simulink model "LM_TOS_new"  (R2018b)
settings: Solver=FixedStepDiscrete  StartTime=0.0  StopTime=inf  FixedStep=0.005  RelTol=1e-3
PostLoadFcn:
  | if any(exist('dsrtsu_mdlpostloadfcn', 'file') ~= 0), dsrtsu_mdlpostloadfcn('Execute', bdroot); end
libraries: rtican x35
(part 10 of 11)

== system LM_TOS_new/LM_TOS_MODEL/adapter2/Lane_2/Subsystem13 ==
  <LANE_2_TARGETOBJECT_0_ST> : Inport
  Bus Creator1 : BusCreator  Inputs=7  OutDataTypeStr=Bus: SEGMENT  NonVirtualBus=on
  Bus Selector4 : BusSelector  OutputSignals=coef_arr_f_0,coef_arr_f_1,coef_arr_f_2,coef_arr_f_3,dlowerLimit_f,dupperLimit_f,numOfSegment_un8,available_b,detectedByVideo_b,quality_f
  Vector Concatenate : Concatenate  NumInputs=4
  SEGMENT_ST : Outport  OutDataTypeStr=Bus: SEGMENT
  wires:
  Bus Selector4/6 -> Bus Creator1/3  "<dupperLimit_f>"
  Bus Selector4/7 -> Bus Creator1/4  "<numOfSegment_un8>"
  Bus Selector4/8 -> Bus Creator1/5  "<available_b>"
  Bus Selector4/9 -> Bus Creator1/6  "<detectedByVideo_b>"
  Bus Selector4/10 -> Bus Creator1/7  "<quality_f>"
  Bus Selector4/5 -> Bus Creator1/2  "<dlowerLimit_f>"
  Vector Concatenate/1 -> Bus Creator1/1
  Bus Selector4/4 -> Vector Concatenate/4  "<coef_arr_f_3>"
  Bus Selector4/3 -> Vector Concatenate/3  "<coef_arr_f_2>"
  Bus Selector4/1 -> Vector Concatenate/1  "<coef_arr_f_0>"
  Bus Selector4/2 -> Vector Concatenate/2  "<coef_arr_f_1>"
  <LANE_2_TARGETOBJECT_0_ST>/1 -> Bus Selector4/1
  Bus Creator1/1 -> SEGMENT_ST/1

== system LM_TOS_new/LM_TOS_MODEL/adapter2/Lane_2/Subsystem14 ==
  <LANE_2_TARGETOBJECT_0_ST> : Inport
  Bus Creator1 : BusCreator  Inputs=7  OutDataTypeStr=Bus: SEGMENT  NonVirtualBus=on
  Bus Selector4 : BusSelector  OutputSignals=coef_arr_f_0,coef_arr_f_1,coef_arr_f_2,coef_arr_f_3,dlowerLimit_f,dupperLimit_f,numOfSegment_un8,available_b,detectedByVideo_b,quality_f
  Vector Concatenate : Concatenate  NumInputs=4
  SEGMENT_ST : Outport  OutDataTypeStr=Bus: SEGMENT
  wires:
  Bus Creator1/1 -> SEGMENT_ST/1
  <LANE_2_TARGETOBJECT_0_ST>/1 -> Bus Selector4/1
  Bus Selector4/2 -> Vector Concatenate/2  "<coef_arr_f_1>"
  Bus Selector4/1 -> Vector Concatenate/1  "<coef_arr_f_0>"
  Bus Selector4/3 -> Vector Concatenate/3  "<coef_arr_f_2>"
  Bus Selector4/4 -> Vector Concatenate/4  "<coef_arr_f_3>"
  Vector Concatenate/1 -> Bus Creator1/1
  Bus Selector4/5 -> Bus Creator1/2  "<dlowerLimit_f>"
  Bus Selector4/10 -> Bus Creator1/7  "<quality_f>"
  Bus Selector4/9 -> Bus Creator1/6  "<detectedByVideo_b>"
  Bus Selector4/8 -> Bus Creator1/5  "<available_b>"
  Bus Selector4/7 -> Bus Creator1/4  "<numOfSegment_un8>"
  Bus Selector4/6 -> Bus Creator1/3  "<dupperLimit_f>"

== system LM_TOS_new/LM_TOS_MODEL/adapter2/Lane_2/Subsystem15 ==
  <LANE_2_TARGETOBJECT_0_ST> : Inport
  Bus Creator1 : BusCreator  Inputs=7  OutDataTypeStr=Bus: SEGMENT  NonVirtualBus=on
  Bus Selector4 : BusSelector  OutputSignals=coef_arr_f_0,coef_arr_f_1,coef_arr_f_2,coef_arr_f_3,dlowerLimit_f,dupperLimit_f,numOfSegment_un8,available_b,detectedByVideo_b,quality_f
  Vector Concatenate : Concatenate  NumInputs=4
  SEGMENT_ST : Outport  OutDataTypeStr=Bus: SEGMENT
  wires:
  Bus Selector4/6 -> Bus Creator1/3  "<dupperLimit_f>"
  Bus Selector4/7 -> Bus Creator1/4  "<numOfSegment_un8>"
  Bus Selector4/8 -> Bus Creator1/5  "<available_b>"
  Bus Selector4/9 -> Bus Creator1/6  "<detectedByVideo_b>"
  Bus Selector4/10 -> Bus Creator1/7  "<quality_f>"
  Bus Selector4/5 -> Bus Creator1/2  "<dlowerLimit_f>"
  Vector Concatenate/1 -> Bus Creator1/1
  Bus Selector4/4 -> Vector Concatenate/4  "<coef_arr_f_3>"
  Bus Selector4/3 -> Vector Concatenate/3  "<coef_arr_f_2>"
  Bus Selector4/1 -> Vector Concatenate/1  "<coef_arr_f_0>"
  Bus Selector4/2 -> Vector Concatenate/2  "<coef_arr_f_1>"
  <LANE_2_TARGETOBJECT_0_ST>/1 -> Bus Selector4/1
  Bus Creator1/1 -> SEGMENT_ST/1

== system LM_TOS_new/LM_TOS_MODEL/adapter2/Lane_2/Subsystem2 ==
  <LANE_0_TARGETOBJECT_0_ST> : Inport
  Bus Creator1 : BusCreator  Inputs=9  OutDataTypeStr=Bus: TARGETOBJECT  NonVirtualBus=on
  Bus Selector4 : BusSelector  OutputSignals=dis2EgoLaneCenter,TTC_f,ID_un8,Index_un8,probWithinLane_arr_f_0,probWithinLane_arr_f_1,probWithinLane_arr_f_2,probWithinLane_arr_f_3,probWithinLane_arr_f_4,probCutIn_f,probCutOut_f,overlap_f,trackingTimeWithinLane_f
  Vector Concatenate : Concatenate  NumInputs=5
  TARGRTOBJECTS_ST : Outport  OutDataTypeStr=Bus: TARGETOBJECT
  wires:
  Bus Selector4/4 -> Bus Creator1/4  "<Index_un8>"
  Bus Creator1/1 -> TARGRTOBJECTS_ST/1
  Bus Selector4/3 -> Bus Creator1/3  "<ID_un8>"
  Vector Concatenate/1 -> Bus Creator1/5
  Bus Selector4/7 -> Vector Concatenate/3  "<probWithinLane_arr_f_2>"
  Bus Selector4/1 -> Bus Creator1/1  "<dis2EgoLaneCenter>"
  Bus Selector4/13 -> Bus Creator1/9  "<trackingTimeWithinLane_f>"
  Bus Selector4/6 -> Vector Concatenate/2  "<probWithinLane_arr_f_1>"
  <LANE_0_TARGETOBJECT_0_ST>/1 -> Bus Selector4/1
  Bus Selector4/5 -> Vector Concatenate/1  "<probWithinLane_arr_f_0>"
  Bus Selector4/2 -> Bus Creator1/2  "<TTC_f>"
  Bus Selector4/9 -> Vector Concatenate/5  "<probWithinLane_arr_f_4>"
  Bus Selector4/12 -> Bus Creator1/8  "<overlap_f>"
  Bus Selector4/10 -> Bus Creator1/6  "<probCutIn_f>"
  Bus Selector4/11 -> Bus Creator1/7  "<probCutOut_f>"
  Bus Selector4/8 -> Vector Concatenate/4  "<probWithinLane_arr_f_3>"

== system LM_TOS_new/LM_TOS_MODEL/adapter2/Lane_2/Subsystem3 ==
  <LANE_0_TARGETOBJECT_0_ST> : Inport
  Bus Creator1 : BusCreator  Inputs=9  OutDataTypeStr=Bus: TARGETOBJECT  NonVirtualBus=on
  Bus Selector4 : BusSelector  OutputSignals=dis2EgoLaneCenter,TTC_f,ID_un8,Index_un8,probWithinLane_arr_f_0,probWithinLane_arr_f_1,probWithinLane_arr_f_2,probWithinLane_arr_f_3,probWithinLane_arr_f_4,probCutIn_f,probCutOut_f,overlap_f,trackingTimeWithinLane_f
  Vector Concatenate : Concatenate  NumInputs=5
  TARGRTOBJECTS_ST : Outport  OutDataTypeStr=Bus: TARGETOBJECT
  wires:
  Bus Selector4/8 -> Vector Concatenate/4  "<probWithinLane_arr_f_3>"
  Bus Selector4/11 -> Bus Creator1/7  "<probCutOut_f>"
  Bus Selector4/10 -> Bus Creator1/6  "<probCutIn_f>"
  Bus Selector4/12 -> Bus Creator1/8  "<overlap_f>"
  Bus Selector4/9 -> Vector Concatenate/5  "<probWithinLane_arr_f_4>"
  Bus Selector4/2 -> Bus Creator1/2  "<TTC_f>"
  Bus Selector4/5 -> Vector Concatenate/1  "<probWithinLane_arr_f_0>"
  <LANE_0_TARGETOBJECT_0_ST>/1 -> Bus Selector4/1
  Bus Selector4/6 -> Vector Concatenate/2  "<probWithinLane_arr_f_1>"
  Bus Selector4/13 -> Bus Creator1/9  "<trackingTimeWithinLane_f>"
  Bus Selector4/1 -> Bus Creator1/1  "<dis2EgoLaneCenter>"
  Bus Selector4/7 -> Vector Concatenate/3  "<probWithinLane_arr_f_2>"
  Vector Concatenate/1 -> Bus Creator1/5
  Bus Selector4/3 -> Bus Creator1/3  "<ID_un8>"
  Bus Creator1/1 -> TARGRTOBJECTS_ST/1
  Bus Selector4/4 -> Bus Creator1/4  "<Index_un8>"

== system LM_TOS_new/LM_TOS_MODEL/adapter2/Lane_2/Subsystem4 ==
  <LANE_0_TARGETOBJECT_0_ST> : Inport
  Bus Creator1 : BusCreator  Inputs=9  OutDataTypeStr=Bus: TARGETOBJECT  NonVirtualBus=on
  Bus Selector4 : BusSelector  OutputSignals=dis2EgoLaneCenter,TTC_f,ID_un8,Index_un8,probWithinLane_arr_f_0,probWithinLane_arr_f_1,probWithinLane_arr_f_2,probWithinLane_arr_f_3,probWithinLane_arr_f_4,probCutIn_f,probCutOut_f,overlap_f,trackingTimeWithinLane_f
  Vector Concatenate : Concatenate  NumInputs=5
  TARGRTOBJECTS_ST : Outport  OutDataTypeStr=Bus: TARGETOBJECT
  wires:
  Bus Selector4/4 -> Bus Creator1/4  "<Index_un8>"
  Bus Creator1/1 -> TARGRTOBJECTS_ST/1
  Bus Selector4/3 -> Bus Creator1/3  "<ID_un8>"
  Vector Concatenate/1 -> Bus Creator1/5
  Bus Selector4/7 -> Vector Concatenate/3  "<probWithinLane_arr_f_2>"
  Bus Selector4/1 -> Bus Creator1/1  "<dis2EgoLaneCenter>"
  Bus Selector4/13 -> Bus Creator1/9  "<trackingTimeWithinLane_f>"
  Bus Selector4/6 -> Vector Concatenate/2  "<probWithinLane_arr_f_1>"
  <LANE_0_TARGETOBJECT_0_ST>/1 -> Bus Selector4/1
  Bus Selector4/5 -> Vector Concatenate/1  "<probWithinLane_arr_f_0>"
  Bus Selector4/2 -> Bus Creator1/2  "<TTC_f>"
  Bus Selector4/9 -> Vector Concatenate/5  "<probWithinLane_arr_f_4>"
  Bus Selector4/12 -> Bus Creator1/8  "<overlap_f>"
  Bus Selector4/10 -> Bus Creator1/6  "<probCutIn_f>"
  Bus Selector4/11 -> Bus Creator1/7  "<probCutOut_f>"
  Bus Selector4/8 -> Vector Concatenate/4  "<probWithinLane_arr_f_3>"

== system LM_TOS_new/LM_TOS_MODEL/adapter2/Lane_2/Subsystem5 ==
  <LANE_0_TARGETOBJECT_0_ST> : Inport
  Bus Creator1 : BusCreator  Inputs=9  OutDataTypeStr=Bus: TARGETOBJECT  NonVirtualBus=on
  Bus Selector4 : BusSelector  OutputSignals=dis2EgoLaneCenter,TTC_f,ID_un8,Index_un8,probWithinLane_arr_f_0,probWithinLane_arr_f_1,probWithinLane_arr_f_2,probWithinLane_arr_f_3,probWithinLane_arr_f_4,probCutIn_f,probCutOut_f,overlap_f,trackingTimeWithinLane_f
  Vector Concatenate : Concatenate  NumInputs=5
  TARGRTOBJECTS_ST : Outport  OutDataTypeStr=Bus: TARGETOBJECT
  wires:
  Bus Selector4/8 -> Vector Concatenate/4  "<probWithinLane_arr_f_3>"
  Bus Selector4/11 -> Bus Creator1/7  "<probCutOut_f>"
  Bus Selector4/10 -> Bus Creator1/6  "<probCutIn_f>"
  Bus Selector4/12 -> Bus Creator1/8  "<overlap_f>"
  Bus Selector4/9 -> Vector Concatenate/5  "<probWithinLane_arr_f_4>"
  Bus Selector4/2 -> Bus Creator1/2  "<TTC_f>"
  Bus Selector4/5 -> Vector Concatenate/1  "<probWithinLane_arr_f_0>"
  <LANE_0_TARGETOBJECT_0_ST>/1 -> Bus Selector4/1
  Bus Selector4/6 -> Vector Concatenate/2  "<probWithinLane_arr_f_1>"
  Bus Selector4/13 -> Bus Creator1/9  "<trackingTimeWithinLane_f>"
  Bus Selector4/1 -> Bus Creator1/1  "<dis2EgoLaneCenter>"
  Bus Selector4/7 -> Vector Concatenate/3  "<probWithinLane_arr_f_2>"
  Vector Concatenate/1 -> Bus Creator1/5
  Bus Selector4/3 -> Bus Creator1/3  "<ID_un8>"
  Bus Creator1/1 -> TARGRTOBJECTS_ST/1
  Bus Selector4/4 -> Bus Creator1/4  "<Index_un8>"

== system LM_TOS_new/LM_TOS_MODEL/adapter2/Lane_2/Subsystem6 ==
  <LANE_0_TARGETOBJECT_0_ST> : Inport
  Bus Creator1 : BusCreator  Inputs=9  OutDataTypeStr=Bus: TARGETOBJECT  NonVirtualBus=on
  Bus Selector4 : BusSelector  OutputSignals=dis2EgoLaneCenter,TTC_f,ID_un8,Index_un8,probWithinLane_arr_f_0,probWithinLane_arr_f_1,probWithinLane_arr_f_2,probWithinLane_arr_f_3,probWithinLane_arr_f_4,probCutIn_f,probCutOut_f,overlap_f,trackingTimeWithinLane_f
  Vector Concatenate : Concatenate  NumInputs=5
  TARGRTOBJECTS_ST : Outport  OutDataTypeStr=Bus: TARGETOBJECT
  wires:
  Bus Selector4/4 -> Bus Creator1/4  "<Index_un8>"
  Bus Creator1/1 -> TARGRTOBJECTS_ST/1
  Bus Selector4/3 -> Bus Creator1/3  "<ID_un8>"
  Vector Concatenate/1 -> Bus Creator1/5
  Bus Selector4/7 -> Vector Concatenate/3  "<probWithinLane_arr_f_2>"
  Bus Selector4/1 -> Bus Creator1/1  "<dis2EgoLaneCenter>"
  Bus Selector4/13 -> Bus Creator1/9  "<trackingTimeWithinLane_f>"
  Bus Selector4/6 -> Vector Concatenate/2  "<probWithinLane_arr_f_1>"
  <LANE_0_TARGETOBJECT_0_ST>/1 -> Bus Selector4/1
  Bus Selector4/5 -> Vector Concatenate/1  "<probWithinLane_arr_f_0>"
  Bus Selector4/2 -> Bus Creator1/2  "<TTC_f>"
  Bus Selector4/9 -> Vector Concatenate/5  "<probWithinLane_arr_f_4>"
  Bus Selector4/12 -> Bus Creator1/8  "<overlap_f>"
  Bus Selector4/10 -> Bus Creator1/6  "<probCutIn_f>"
  Bus Selector4/11 -> Bus Creator1/7  "<probCutOut_f>"
  Bus Selector4/8 -> Vector Concatenate/4  "<probWithinLane_arr_f_3>"

== system LM_TOS_new/LM_TOS_MODEL/adapter2/Lane_2/Subsystem7 ==
  <LANE_0_TARGETOBJECT_0_ST> : Inport
  Bus Creator1 : BusCreator  Inputs=9  OutDataTypeStr=Bus: TARGETOBJECT  NonVirtualBus=on
  Bus Selector4 : BusSelector  OutputSignals=dis2EgoLaneCenter,TTC_f,ID_un8,Index_un8,probWithinLane_arr_f_0,probWithinLane_arr_f_1,probWithinLane_arr_f_2,probWithinLane_arr_f_3,probWithinLane_arr_f_4,probCutIn_f,probCutOut_f,overlap_f,trackingTimeWithinLane_f
  Vector Concatenate : Concatenate  NumInputs=5
  TARGRTOBJECTS_ST : Outport  OutDataTypeStr=Bus: TARGETOBJECT
  wires:
  Bus Selector4/8 -> Vector Concatenate/4  "<probWithinLane_arr_f_3>"
  Bus Selector4/11 -> Bus Creator1/7  "<probCutOut_f>"
  Bus Selector4/10 -> Bus Creator1/6  "<probCutIn_f>"
  Bus Selector4/12 -> Bus Creator1/8  "<overlap_f>"
  Bus Selector4/9 -> Vector Concatenate/5  "<probWithinLane_arr_f_4>"
  Bus Selector4/2 -> Bus Creator1/2  "<TTC_f>"
  Bus Selector4/5 -> Vector Concatenate/1  "<probWithinLane_arr_f_0>"
  <LANE_0_TARGETOBJECT_0_ST>/1 -> Bus Selector4/1
  Bus Selector4/6 -> Vector Concatenate/2  "<probWithinLane_arr_f_1>"
  Bus Selector4/13 -> Bus Creator1/9  "<trackingTimeWithinLane_f>"
  Bus Selector4/1 -> Bus Creator1/1  "<dis2EgoLaneCenter>"
  Bus Selector4/7 -> Vector Concatenate/3  "<probWithinLane_arr_f_2>"
  Vector Concatenate/1 -> Bus Creator1/5
  Bus Selector4/3 -> Bus Creator1/3  "<ID_un8>"
  Bus Creator1/1 -> TARGRTOBJECTS_ST/1
  Bus Selector4/4 -> Bus Creator1/4  "<Index_un8>"

== system LM_TOS_new/LM_TOS_MODEL/adapter2/Lane_2/Subsystem8 ==
  <LANE_0_TARGETOBJECT_0_ST> : Inport
  Bus Creator1 : BusCreator  Inputs=9  OutDataTypeStr=Bus: TARGETOBJECT  NonVirtualBus=on
  Bus Selector4 : BusSelector  OutputSignals=dis2EgoLaneCenter,TTC_f,ID_un8,Index_un8,probWithinLane_arr_f_0,probWithinLane_arr_f_1,probWithinLane_arr_f_2,probWithinLane_arr_f_3,probWithinLane_arr_f_4,probCutIn_f,probCutOut_f,overlap_f,trackingTimeWithinLane_f
  Vector Concatenate : Concatenate  NumInputs=5
  TARGRTOBJECTS_ST : Outport  OutDataTypeStr=Bus: TARGETOBJECT
  wires:
  Bus Selector4/4 -> Bus Creator1/4  "<Index_un8>"
  Bus Creator1/1 -> TARGRTOBJECTS_ST/1
  Bus Selector4/3 -> Bus Creator1/3  "<ID_un8>"
  Vector Concatenate/1 -> Bus Creator1/5
  Bus Selector4/7 -> Vector Concatenate/3  "<probWithinLane_arr_f_2>"
  Bus Selector4/1 -> Bus Creator1/1  "<dis2EgoLaneCenter>"
  Bus Selector4/13 -> Bus Creator1/9  "<trackingTimeWithinLane_f>"
  Bus Selector4/6 -> Vector Concatenate/2  "<probWithinLane_arr_f_1>"
  <LANE_0_TARGETOBJECT_0_ST>/1 -> Bus Selector4/1
  Bus Selector4/5 -> Vector Concatenate/1  "<probWithinLane_arr_f_0>"
  Bus Selector4/2 -> Bus Creator1/2  "<TTC_f>"
  Bus Selector4/9 -> Vector Concatenate/5  "<probWithinLane_arr_f_4>"
  Bus Selector4/12 -> Bus Creator1/8  "<overlap_f>"
  Bus Selector4/10 -> Bus Creator1/6  "<probCutIn_f>"
  Bus Selector4/11 -> Bus Creator1/7  "<probCutOut_f>"
  Bus Selector4/8 -> Vector Concatenate/4  "<probWithinLane_arr_f_3>"

== system LM_TOS_new/LM_TOS_MODEL/adapter2/Lane_2/Subsystem9 ==
  <LANE_0_TARGETOBJECT_0_ST> : Inport
  Bus Creator1 : BusCreator  Inputs=9  OutDataTypeStr=Bus: TARGETOBJECT  NonVirtualBus=on
  Bus Selector4 : BusSelector  OutputSignals=dis2EgoLaneCenter,TTC_f,ID_un8,Index_un8,probWithinLane_arr_f_0,probWithinLane_arr_f_1,probWithinLane_arr_f_2,probWithinLane_arr_f_3,probWithinLane_arr_f_4,probCutIn_f,probCutOut_f,overlap_f,trackingTimeWithinLane_f
  Vector Concatenate : Concatenate  NumInputs=5
  TARGRTOBJECTS_ST : Outport  OutDataTypeStr=Bus: TARGETOBJECT
  wires:
  Bus Selector4/8 -> Vector Concatenate/4  "<probWithinLane_arr_f_3>"
  Bus Selector4/11 -> Bus Creator1/7  "<probCutOut_f>"
  Bus Selector4/10 -> Bus Creator1/6  "<probCutIn_f>"
  Bus Selector4/12 -> Bus Creator1/8  "<overlap_f>"
  Bus Selector4/9 -> Vector Concatenate/5  "<probWithinLane_arr_f_4>"
  Bus Selector4/2 -> Bus Creator1/2  "<TTC_f>"
  Bus Selector4/5 -> Vector Concatenate/1  "<probWithinLane_arr_f_0>"
  <LANE_0_TARGETOBJECT_0_ST>/1 -> Bus Selector4/1
  Bus Selector4/6 -> Vector Concatenate/2  "<probWithinLane_arr_f_1>"
  Bus Selector4/13 -> Bus Creator1/9  "<trackingTimeWithinLane_f>"
  Bus Selector4/1 -> Bus Creator1/1  "<dis2EgoLaneCenter>"
  Bus Selector4/7 -> Vector Concatenate/3  "<probWithinLane_arr_f_2>"
  Vector Concatenate/1 -> Bus Creator1/5
  Bus Selector4/3 -> Bus Creator1/3  "<ID_un8>"
  Bus Creator1/1 -> TARGRTOBJECTS_ST/1
  Bus Selector4/4 -> Bus Creator1/4  "<Index_un8>"

== system LM_TOS_new/LM_TOS_MODEL/adapter2/Lane_3/Subsystem ==
  <LANE_3_TARGETOBJECT_0_ST> : Inport
  Bus Creator1 : BusCreator  Inputs=9  OutDataTypeStr=Bus: TARGETOBJECT  NonVirtualBus=on
  Bus Selector4 : BusSelector  OutputSignals=dis2EgoLaneCenter,TTC_f,ID_un8,Index_un8,probWithinLane_arr_f_0,probWithinLane_arr_f_1,probWithinLane_arr_f_2,probWithinLane_arr_f_3,probWithinLane_arr_f_4,probCutIn_f,probCutOut_f,overlap_f,trackingTimeWithinLane_f
  Vector Concatenate : Concatenate  NumInputs=5
  TARGRTOBJECTS_ST : Outport  OutDataTypeStr=Bus: TARGETOBJECT
  wires:
  Bus Selector4/8 -> Vector Concatenate/4  "<probWithinLane_arr_f_3>"
  Bus Selector4/11 -> Bus Creator1/7  "<probCutOut_f>"
  Bus Selector4/10 -> Bus Creator1/6  "<probCutIn_f>"
  Bus Selector4/12 -> Bus Creator1/8  "<overlap_f>"
  Bus Selector4/9 -> Vector Concatenate/5  "<probWithinLane_arr_f_4>"
  Bus Selector4/2 -> Bus Creator1/2  "<TTC_f>"
  Bus Selector4/5 -> Vector Concatenate/1  "<probWithinLane_arr_f_0>"
  <LANE_3_TARGETOBJECT_0_ST>/1 -> Bus Selector4/1
  Bus Selector4/6 -> Vector Concatenate/2  "<probWithinLane_arr_f_1>"
  Bus Selector4/13 -> Bus Creator1/9  "<trackingTimeWithinLane_f>"
  Bus Selector4/1 -> Bus Creator1/1  "<dis2EgoLaneCenter>"
  Bus Selector4/7 -> Vector Concatenate/3  "<probWithinLane_arr_f_2>"
  Vector Concatenate/1 -> Bus Creator1/5
  Bus Selector4/3 -> Bus Creator1/3  "<ID_un8>"
  Bus Creator1/1 -> TARGRTOBJECTS_ST/1
  Bus Selector4/4 -> Bus Creator1/4  "<Index_un8>"

== system LM_TOS_new/LM_TOS_MODEL/adapter2/Lane_3/Subsystem1 ==
  <LANE_3_TARGETOBJECT_0_ST> : Inport
  Bus Creator1 : BusCreator  Inputs=9  OutDataTypeStr=Bus: TARGETOBJECT  NonVirtualBus=on
  Bus Selector4 : BusSelector  OutputSignals=dis2EgoLaneCenter,TTC_f,ID_un8,Index_un8,probWithinLane_arr_f_0,probWithinLane_arr_f_1,probWithinLane_arr_f_2,probWithinLane_arr_f_3,probWithinLane_arr_f_4,probCutIn_f,probCutOut_f,overlap_f,trackingTimeWithinLane_f
  Vector Concatenate : Concatenate  NumInputs=5
  TARGRTOBJECTS_ST : Outport  OutDataTypeStr=Bus: TARGETOBJECT
  wires:
  Bus Selector4/4 -> Bus Creator1/4  "<Index_un8>"
  Bus Creator1/1 -> TARGRTOBJECTS_ST/1
  Bus Selector4/3 -> Bus Creator1/3  "<ID_un8>"
  Vector Concatenate/1 -> Bus Creator1/5
  Bus Selector4/7 -> Vector Concatenate/3  "<probWithinLane_arr_f_2>"
  Bus Selector4/1 -> Bus Creator1/1  "<dis2EgoLaneCenter>"
  Bus Selector4/13 -> Bus Creator1/9  "<trackingTimeWithinLane_f>"
  Bus Selector4/6 -> Vector Concatenate/2  "<probWithinLane_arr_f_1>"
  <LANE_3_TARGETOBJECT_0_ST>/1 -> Bus Selector4/1
  Bus Selector4/5 -> Vector Concatenate/1  "<probWithinLane_arr_f_0>"
  Bus Selector4/2 -> Bus Creator1/2  "<TTC_f>"
  Bus Selector4/9 -> Vector Concatenate/5  "<probWithinLane_arr_f_4>"
  Bus Selector4/12 -> Bus Creator1/8  "<overlap_f>"
  Bus Selector4/10 -> Bus Creator1/6  "<probCutIn_f>"
  Bus Selector4/11 -> Bus Creator1/7  "<probCutOut_f>"
  Bus Selector4/8 -> Vector Concatenate/4  "<probWithinLane_arr_f_3>"

== system LM_TOS_new/LM_TOS_MODEL/adapter2/Lane_3/Subsystem10 ==
  <LANE_3_TARGETOBJECT_0_ST> : Inport
  Bus Creator1 : BusCreator  Inputs=7  OutDataTypeStr=Bus: SEGMENT  NonVirtualBus=on
  Bus Selector4 : BusSelector  OutputSignals=coef_arr_f_0,coef_arr_f_1,coef_arr_f_2,coef_arr_f_3,dlowerLimit_f,dupperLimit_f,numOfSegment_un8,available_b,detectedByVideo_b,quality_f
  Vector Concatenate : Concatenate  NumInputs=4
  SEGMENT_ST : Outport  OutDataTypeStr=Bus: SEGMENT
  wires:
  Bus Selector4/6 -> Bus Creator1/3  "<dupperLimit_f>"
  Bus Selector4/7 -> Bus Creator1/4  "<numOfSegment_un8>"
  Bus Selector4/8 -> Bus Creator1/5  "<available_b>"
  Bus Selector4/9 -> Bus Creator1/6  "<detectedByVideo_b>"
  Bus Selector4/10 -> Bus Creator1/7  "<quality_f>"
  Bus Selector4/5 -> Bus Creator1/2  "<dlowerLimit_f>"
  Vector Concatenate/1 -> Bus Creator1/1
  Bus Selector4/4 -> Vector Concatenate/4  "<coef_arr_f_3>"
  Bus Selector4/3 -> Vector Concatenate/3  "<coef_arr_f_2>"
  Bus Selector4/1 -> Vector Concatenate/1  "<coef_arr_f_0>"
  Bus Selector4/2 -> Vector Concatenate/2  "<coef_arr_f_1>"
  <LANE_3_TARGETOBJECT_0_ST>/1 -> Bus Selector4/1
  Bus Creator1/1 -> SEGMENT_ST/1

== system LM_TOS_new/LM_TOS_MODEL/adapter2/Lane_3/Subsystem11 ==
  <LANE_3_TARGETOBJECT_0_ST> : Inport
  Bus Creator1 : BusCreator  Inputs=7  OutDataTypeStr=Bus: SEGMENT  NonVirtualBus=on
  Bus Selector4 : BusSelector  OutputSignals=coef_arr_f_0,coef_arr_f_1,coef_arr_f_2,coef_arr_f_3,dlowerLimit_f,dupperLimit_f,numOfSegment_un8,available_b,detectedByVideo_b,quality_f
  Vector Concatenate : Concatenate  NumInputs=4
  SEGMENT_ST : Outport  OutDataTypeStr=Bus: SEGMENT
  wires:
  Bus Creator1/1 -> SEGMENT_ST/1
  <LANE_3_TARGETOBJECT_0_ST>/1 -> Bus Selector4/1
  Bus Selector4/2 -> Vector Concatenate/2  "<coef_arr_f_1>"
  Bus Selector4/1 -> Vector Concatenate/1  "<coef_arr_f_0>"
  Bus Selector4/3 -> Vector Concatenate/3  "<coef_arr_f_2>"
  Bus Selector4/4 -> Vector Concatenate/4  "<coef_arr_f_3>"
  Vector Concatenate/1 -> Bus Creator1/1
  Bus Selector4/5 -> Bus Creator1/2  "<dlowerLimit_f>"
  Bus Selector4/10 -> Bus Creator1/7  "<quality_f>"
  Bus Selector4/9 -> Bus Creator1/6  "<detectedByVideo_b>"
  Bus Selector4/8 -> Bus Creator1/5  "<available_b>"
  Bus Selector4/7 -> Bus Creator1/4  "<numOfSegment_un8>"
  Bus Selector4/6 -> Bus Creator1/3  "<dupperLimit_f>"

== system LM_TOS_new/LM_TOS_MODEL/adapter2/Lane_3/Subsystem12 ==
  <LANE_3_TARGETOBJECT_0_ST> : Inport
  Bus Creator1 : BusCreator  Inputs=7  OutDataTypeStr=Bus: SEGMENT  NonVirtualBus=on
  Bus Selector4 : BusSelector  OutputSignals=coef_arr_f_0,coef_arr_f_1,coef_arr_f_2,coef_arr_f_3,dlowerLimit_f,dupperLimit_f,numOfSegment_un8,available_b,detectedByVideo_b,quality_f
  Vector Concatenate : Concatenate  NumInputs=4
  SEGMENT_ST : Outport  OutDataTypeStr=Bus: SEGMENT
  wires:
  Bus Selector4/6 -> Bus Creator1/3  "<dupperLimit_f>"
  Bus Selector4/7 -> Bus Creator1/4  "<numOfSegment_un8>"
  Bus Selector4/8 -> Bus Creator1/5  "<available_b>"
  Bus Selector4/9 -> Bus Creator1/6  "<detectedByVideo_b>"
  Bus Selector4/10 -> Bus Creator1/7  "<quality_f>"
  Bus Selector4/5 -> Bus Creator1/2  "<dlowerLimit_f>"
  Vector Concatenate/1 -> Bus Creator1/1
  Bus Selector4/4 -> Vector Concatenate/4  "<coef_arr_f_3>"
  Bus Selector4/3 -> Vector Concatenate/3  "<coef_arr_f_2>"
  Bus Selector4/1 -> Vector Concatenate/1  "<coef_arr_f_0>"
  Bus Selector4/2 -> Vector Concatenate/2  "<coef_arr_f_1>"
  <LANE_3_TARGETOBJECT_0_ST>/1 -> Bus Selector4/1
  Bus Creator1/1 -> SEGMENT_ST/1

== system LM_TOS_new/LM_TOS_MODEL/adapter2/Lane_3/Subsystem13 ==
  <LANE_3_TARGETOBJECT_0_ST> : Inport
  Bus Creator1 : BusCreator  Inputs=7  OutDataTypeStr=Bus: SEGMENT  NonVirtualBus=on
  Bus Selector4 : BusSelector  OutputSignals=coef_arr_f_0,coef_arr_f_1,coef_arr_f_2,coef_arr_f_3,dlowerLimit_f,dupperLimit_f,numOfSegment_un8,available_b,detectedByVideo_b,quality_f
  Vector Concatenate : Concatenate  NumInputs=4
  SEGMENT_ST : Outport  OutDataTypeStr=Bus: SEGMENT
  wires:
  Bus Creator1/1 -> SEGMENT_ST/1
  <LANE_3_TARGETOBJECT_0_ST>/1 -> Bus Selector4/1
  Bus Selector4/2 -> Vector Concatenate/2  "<coef_arr_f_1>"
  Bus Selector4/1 -> Vector Concatenate/1  "<coef_arr_f_0>"
  Bus Selector4/3 -> Vector Concatenate/3  "<coef_arr_f_2>"
  Bus Selector4/4 -> Vector Concatenate/4  "<coef_arr_f_3>"
  Vector Concatenate/1 -> Bus Creator1/1
  Bus Selector4/5 -> Bus Creator1/2  "<dlowerLimit_f>"
  Bus Selector4/10 -> Bus Creator1/7  "<quality_f>"
  Bus Selector4/9 -> Bus Creator1/6  "<detectedByVideo_b>"
  Bus Selector4/8 -> Bus Creator1/5  "<available_b>"
  Bus Selector4/7 -> Bus Creator1/4  "<numOfSegment_un8>"
  Bus Selector4/6 -> Bus Creator1/3  "<dupperLimit_f>"

== system LM_TOS_new/LM_TOS_MODEL/adapter2/Lane_3/Subsystem14 ==
  <LANE_3_TARGETOBJECT_0_ST> : Inport
  Bus Creator1 : BusCreator  Inputs=7  OutDataTypeStr=Bus: SEGMENT  NonVirtualBus=on
  Bus Selector4 : BusSelector  OutputSignals=coef_arr_f_0,coef_arr_f_1,coef_arr_f_2,coef_arr_f_3,dlowerLimit_f,dupperLimit_f,numOfSegment_un8,available_b,detectedByVideo_b,quality_f
  Vector Concatenate : Concatenate  NumInputs=4
  SEGMENT_ST : Outport  OutDataTypeStr=Bus: SEGMENT
  wires:
  Bus Selector4/6 -> Bus Creator1/3  "<dupperLimit_f>"
  Bus Selector4/7 -> Bus Creator1/4  "<numOfSegment_un8>"
  Bus Selector4/8 -> Bus Creator1/5  "<available_b>"
  Bus Selector4/9 -> Bus Creator1/6  "<detectedByVideo_b>"
  Bus Selector4/10 -> Bus Creator1/7  "<quality_f>"
  Bus Selector4/5 -> Bus Creator1/2  "<dlowerLimit_f>"
  Vector Concatenate/1 -> Bus Creator1/1
  Bus Selector4/4 -> Vector Concatenate/4  "<coef_arr_f_3>"
  Bus Selector4/3 -> Vector Concatenate/3  "<coef_arr_f_2>"
  Bus Selector4/1 -> Vector Concatenate/1  "<coef_arr_f_0>"
  Bus Selector4/2 -> Vector Concatenate/2  "<coef_arr_f_1>"
  <LANE_3_TARGETOBJECT_0_ST>/1 -> Bus Selector4/1
  Bus Creator1/1 -> SEGMENT_ST/1

== system LM_TOS_new/LM_TOS_MODEL/adapter2/Lane_3/Subsystem15 ==
  <LANE_3_TARGETOBJECT_0_ST> : Inport
  Bus Creator1 : BusCreator  Inputs=7  OutDataTypeStr=Bus: SEGMENT  NonVirtualBus=on
  Bus Selector4 : BusSelector  OutputSignals=coef_arr_f_0,coef_arr_f_1,coef_arr_f_2,coef_arr_f_3,dlowerLimit_f,dupperLimit_f,numOfSegment_un8,available_b,detectedByVideo_b,quality_f
  Vector Concatenate : Concatenate  NumInputs=4
  SEGMENT_ST : Outport  OutDataTypeStr=Bus: SEGMENT
  wires:
  Bus Creator1/1 -> SEGMENT_ST/1
  <LANE_3_TARGETOBJECT_0_ST>/1 -> Bus Selector4/1
  Bus Selector4/2 -> Vector Concatenate/2  "<coef_arr_f_1>"
  Bus Selector4/1 -> Vector Concatenate/1  "<coef_arr_f_0>"
  Bus Selector4/3 -> Vector Concatenate/3  "<coef_arr_f_2>"
  Bus Selector4/4 -> Vector Concatenate/4  "<coef_arr_f_3>"
  Vector Concatenate/1 -> Bus Creator1/1
  Bus Selector4/5 -> Bus Creator1/2  "<dlowerLimit_f>"
  Bus Selector4/10 -> Bus Creator1/7  "<quality_f>"
  Bus Selector4/9 -> Bus Creator1/6  "<detectedByVideo_b>"
  Bus Selector4/8 -> Bus Creator1/5  "<available_b>"
  Bus Selector4/7 -> Bus Creator1/4  "<numOfSegment_un8>"
  Bus Selector4/6 -> Bus Creator1/3  "<dupperLimit_f>"

== system LM_TOS_new/LM_TOS_MODEL/adapter2/Lane_3/Subsystem2 ==
  <LANE_3_TARGETOBJECT_0_ST> : Inport
  Bus Creator1 : BusCreator  Inputs=9  OutDataTypeStr=Bus: TARGETOBJECT  NonVirtualBus=on
  Bus Selector4 : BusSelector  OutputSignals=dis2EgoLaneCenter,TTC_f,ID_un8,Index_un8,probWithinLane_arr_f_0,probWithinLane_arr_f_1,probWithinLane_arr_f_2,probWithinLane_arr_f_3,probWithinLane_arr_f_4,probCutIn_f,probCutOut_f,overlap_f,trackingTimeWithinLane_f
  Vector Concatenate : Concatenate  NumInputs=5
  TARGRTOBJECTS_ST : Outport  OutDataTypeStr=Bus: TARGETOBJECT
  wires:
  Bus Selector4/8 -> Vector Concatenate/4  "<probWithinLane_arr_f_3>"
  Bus Selector4/11 -> Bus Creator1/7  "<probCutOut_f>"
  Bus Selector4/10 -> Bus Creator1/6  "<probCutIn_f>"
  Bus Selector4/12 -> Bus Creator1/8  "<overlap_f>"
  Bus Selector4/9 -> Vector Concatenate/5  "<probWithinLane_arr_f_4>"
  Bus Selector4/2 -> Bus Creator1/2  "<TTC_f>"
  Bus Selector4/5 -> Vector Concatenate/1  "<probWithinLane_arr_f_0>"
  <LANE_3_TARGETOBJECT_0_ST>/1 -> Bus Selector4/1
  Bus Selector4/6 -> Vector Concatenate/2  "<probWithinLane_arr_f_1>"
  Bus Selector4/13 -> Bus Creator1/9  "<trackingTimeWithinLane_f>"
  Bus Selector4/1 -> Bus Creator1/1  "<dis2EgoLaneCenter>"
  Bus Selector4/7 -> Vector Concatenate/3  "<probWithinLane_arr_f_2>"
  Vector Concatenate/1 -> Bus Creator1/5
  Bus Selector4/3 -> Bus Creator1/3  "<ID_un8>"
  Bus Creator1/1 -> TARGRTOBJECTS_ST/1
  Bus Selector4/4 -> Bus Creator1/4  "<Index_un8>"

== system LM_TOS_new/LM_TOS_MODEL/adapter2/Lane_3/Subsystem3 ==
  <LANE_3_TARGETOBJECT_0_ST> : Inport
  Bus Creator1 : BusCreator  Inputs=9  OutDataTypeStr=Bus: TARGETOBJECT  NonVirtualBus=on
  Bus Selector4 : BusSelector  OutputSignals=dis2EgoLaneCenter,TTC_f,ID_un8,Index_un8,probWithinLane_arr_f_0,probWithinLane_arr_f_1,probWithinLane_arr_f_2,probWithinLane_arr_f_3,probWithinLane_arr_f_4,probCutIn_f,probCutOut_f,overlap_f,trackingTimeWithinLane_f
  Vector Concatenate : Concatenate  NumInputs=5
  TARGRTOBJECTS_ST : Outport  OutDataTypeStr=Bus: TARGETOBJECT
  wires:
  Bus Selector4/4 -> Bus Creator1/4  "<Index_un8>"
  Bus Creator1/1 -> TARGRTOBJECTS_ST/1
  Bus Selector4/3 -> Bus Creator1/3  "<ID_un8>"
  Vector Concatenate/1 -> Bus Creator1/5
  Bus Selector4/7 -> Vector Concatenate/3  "<probWithinLane_arr_f_2>"
  Bus Selector4/1 -> Bus Creator1/1  "<dis2EgoLaneCenter>"
  Bus Selector4/13 -> Bus Creator1/9  "<trackingTimeWithinLane_f>"
  Bus Selector4/6 -> Vector Concatenate/2  "<probWithinLane_arr_f_1>"
  <LANE_3_TARGETOBJECT_0_ST>/1 -> Bus Selector4/1
  Bus Selector4/5 -> Vector Concatenate/1  "<probWithinLane_arr_f_0>"
  Bus Selector4/2 -> Bus Creator1/2  "<TTC_f>"
  Bus Selector4/9 -> Vector Concatenate/5  "<probWithinLane_arr_f_4>"
  Bus Selector4/12 -> Bus Creator1/8  "<overlap_f>"
  Bus Selector4/10 -> Bus Creator1/6  "<probCutIn_f>"
  Bus Selector4/11 -> Bus Creator1/7  "<probCutOut_f>"
  Bus Selector4/8 -> Vector Concatenate/4  "<probWithinLane_arr_f_3>"

== system LM_TOS_new/LM_TOS_MODEL/adapter2/Lane_3/Subsystem4 ==
  <LANE_3_TARGETOBJECT_0_ST> : Inport
  Bus Creator1 : BusCreator  Inputs=9  OutDataTypeStr=Bus: TARGETOBJECT  NonVirtualBus=on
  Bus Selector4 : BusSelector  OutputSignals=dis2EgoLaneCenter,TTC_f,ID_un8,Index_un8,probWithinLane_arr_f_0,probWithinLane_arr_f_1,probWithinLane_arr_f_2,probWithinLane_arr_f_3,probWithinLane_arr_f_4,probCutIn_f,probCutOut_f,overlap_f,trackingTimeWithinLane_f
  Vector Concatenate : Concatenate  NumInputs=5
  TARGRTOBJECTS_ST : Outport  OutDataTypeStr=Bus: TARGETOBJECT
  wires:
  Bus Selector4/8 -> Vector Concatenate/4  "<probWithinLane_arr_f_3>"
  Bus Selector4/11 -> Bus Creator1/7  "<probCutOut_f>"
  Bus Selector4/10 -> Bus Creator1/6  "<probCutIn_f>"
  Bus Selector4/12 -> Bus Creator1/8  "<overlap_f>"
  Bus Selector4/9 -> Vector Concatenate/5  "<probWithinLane_arr_f_4>"
  Bus Selector4/2 -> Bus Creator1/2  "<TTC_f>"
  Bus Selector4/5 -> Vector Concatenate/1  "<probWithinLane_arr_f_0>"
  <LANE_3_TARGETOBJECT_0_ST>/1 -> Bus Selector4/1
  Bus Selector4/6 -> Vector Concatenate/2  "<probWithinLane_arr_f_1>"
  Bus Selector4/13 -> Bus Creator1/9  "<trackingTimeWithinLane_f>"
  Bus Selector4/1 -> Bus Creator1/1  "<dis2EgoLaneCenter>"
  Bus Selector4/7 -> Vector Concatenate/3  "<probWithinLane_arr_f_2>"
  Vector Concatenate/1 -> Bus Creator1/5
  Bus Selector4/3 -> Bus Creator1/3  "<ID_un8>"
  Bus Creator1/1 -> TARGRTOBJECTS_ST/1
  Bus Selector4/4 -> Bus Creator1/4  "<Index_un8>"

== system LM_TOS_new/LM_TOS_MODEL/adapter2/Lane_3/Subsystem5 ==
  <LANE_3_TARGETOBJECT_0_ST> : Inport
  Bus Creator1 : BusCreator  Inputs=9  OutDataTypeStr=Bus: TARGETOBJECT  NonVirtualBus=on
  Bus Selector4 : BusSelector  OutputSignals=dis2EgoLaneCenter,TTC_f,ID_un8,Index_un8,probWithinLane_arr_f_0,probWithinLane_arr_f_1,probWithinLane_arr_f_2,probWithinLane_arr_f_3,probWithinLane_arr_f_4,probCutIn_f,probCutOut_f,overlap_f,trackingTimeWithinLane_f
  Vector Concatenate : Concatenate  NumInputs=5
  TARGRTOBJECTS_ST : Outport  OutDataTypeStr=Bus: TARGETOBJECT
  wires:
  Bus Selector4/4 -> Bus Creator1/4  "<Index_un8>"
  Bus Creator1/1 -> TARGRTOBJECTS_ST/1
  Bus Selector4/3 -> Bus Creator1/3  "<ID_un8>"
  Vector Concatenate/1 -> Bus Creator1/5
  Bus Selector4/7 -> Vector Concatenate/3  "<probWithinLane_arr_f_2>"
  Bus Selector4/1 -> Bus Creator1/1  "<dis2EgoLaneCenter>"
  Bus Selector4/13 -> Bus Creator1/9  "<trackingTimeWithinLane_f>"
  Bus Selector4/6 -> Vector Concatenate/2  "<probWithinLane_arr_f_1>"
  <LANE_3_TARGETOBJECT_0_ST>/1 -> Bus Selector4/1
  Bus Selector4/5 -> Vector Concatenate/1  "<probWithinLane_arr_f_0>"
  Bus Selector4/2 -> Bus Creator1/2  "<TTC_f>"
  Bus Selector4/9 -> Vector Concatenate/5  "<probWithinLane_arr_f_4>"
  Bus Selector4/12 -> Bus Creator1/8  "<overlap_f>"
  Bus Selector4/10 -> Bus Creator1/6  "<probCutIn_f>"
  Bus Selector4/11 -> Bus Creator1/7  "<probCutOut_f>"
  Bus Selector4/8 -> Vector Concatenate/4  "<probWithinLane_arr_f_3>"

== system LM_TOS_new/LM_TOS_MODEL/adapter2/Lane_3/Subsystem6 ==
  <LANE_3_TARGETOBJECT_0_ST> : Inport
  Bus Creator1 : BusCreator  Inputs=9  OutDataTypeStr=Bus: TARGETOBJECT  NonVirtualBus=on
  Bus Selector4 : BusSelector  OutputSignals=dis2EgoLaneCenter,TTC_f,ID_un8,Index_un8,probWithinLane_arr_f_0,probWithinLane_arr_f_1,probWithinLane_arr_f_2,probWithinLane_arr_f_3,probWithinLane_arr_f_4,probCutIn_f,probCutOut_f,overlap_f,trackingTimeWithinLane_f
  Vector Concatenate : Concatenate  NumInputs=5
  TARGRTOBJECTS_ST : Outport  OutDataTypeStr=Bus: TARGETOBJECT
  wires:
  Bus Selector4/8 -> Vector Concatenate/4  "<probWithinLane_arr_f_3>"
  Bus Selector4/11 -> Bus Creator1/7  "<probCutOut_f>"
  Bus Selector4/10 -> Bus Creator1/6  "<probCutIn_f>"
  Bus Selector4/12 -> Bus Creator1/8  "<overlap_f>"
  Bus Selector4/9 -> Vector Concatenate/5  "<probWithinLane_arr_f_4>"
  Bus Selector4/2 -> Bus Creator1/2  "<TTC_f>"
  Bus Selector4/5 -> Vector Concatenate/1  "<probWithinLane_arr_f_0>"
  <LANE_3_TARGETOBJECT_0_ST>/1 -> Bus Selector4/1
  Bus Selector4/6 -> Vector Concatenate/2  "<probWithinLane_arr_f_1>"
  Bus Selector4/13 -> Bus Creator1/9  "<trackingTimeWithinLane_f>"
  Bus Selector4/1 -> Bus Creator1/1  "<dis2EgoLaneCenter>"
  Bus Selector4/7 -> Vector Concatenate/3  "<probWithinLane_arr_f_2>"
  Vector Concatenate/1 -> Bus Creator1/5
  Bus Selector4/3 -> Bus Creator1/3  "<ID_un8>"
  Bus Creator1/1 -> TARGRTOBJECTS_ST/1
  Bus Selector4/4 -> Bus Creator1/4  "<Index_un8>"

== system LM_TOS_new/LM_TOS_MODEL/adapter2/Lane_3/Subsystem7 ==
  <LANE_3_TARGETOBJECT_0_ST> : Inport
  Bus Creator1 : BusCreator  Inputs=9  OutDataTypeStr=Bus: TARGETOBJECT  NonVirtualBus=on
  Bus Selector4 : BusSelector  OutputSignals=dis2EgoLaneCenter,TTC_f,ID_un8,Index_un8,probWithinLane_arr_f_0,probWithinLane_arr_f_1,probWithinLane_arr_f_2,probWithinLane_arr_f_3,probWithinLane_arr_f_4,probCutIn_f,probCutOut_f,overlap_f,trackingTimeWithinLane_f
  Vector Concatenate : Concatenate  NumInputs=5
  TARGRTOBJECTS_ST : Outport  OutDataTypeStr=Bus: TARGETOBJECT
  wires:
  Bus Selector4/4 -> Bus Creator1/4  "<Index_un8>"
  Bus Creator1/1 -> TARGRTOBJECTS_ST/1
  Bus Selector4/3 -> Bus Creator1/3  "<ID_un8>"
  Vector Concatenate/1 -> Bus Creator1/5
  Bus Selector4/7 -> Vector Concatenate/3  "<probWithinLane_arr_f_2>"
  Bus Selector4/1 -> Bus Creator1/1  "<dis2EgoLaneCenter>"
  Bus Selector4/13 -> Bus Creator1/9  "<trackingTimeWithinLane_f>"
  Bus Selector4/6 -> Vector Concatenate/2  "<probWithinLane_arr_f_1>"
  <LANE_3_TARGETOBJECT_0_ST>/1 -> Bus Selector4/1
  Bus Selector4/5 -> Vector Concatenate/1  "<probWithinLane_arr_f_0>"
  Bus Selector4/2 -> Bus Creator1/2  "<TTC_f>"
  Bus Selector4/9 -> Vector Concatenate/5  "<probWithinLane_arr_f_4>"
  Bus Selector4/12 -> Bus Creator1/8  "<overlap_f>"
  Bus Selector4/10 -> Bus Creator1/6  "<probCutIn_f>"
  Bus Selector4/11 -> Bus Creator1/7  "<probCutOut_f>"
  Bus Selector4/8 -> Vector Concatenate/4  "<probWithinLane_arr_f_3>"

== system LM_TOS_new/LM_TOS_MODEL/adapter2/Lane_3/Subsystem8 ==
  <LANE_3_TARGETOBJECT_0_ST> : Inport
  Bus Creator1 : BusCreator  Inputs=9  OutDataTypeStr=Bus: TARGETOBJECT  NonVirtualBus=on
  Bus Selector4 : BusSelector  OutputSignals=dis2EgoLaneCenter,TTC_f,ID_un8,Index_un8,probWithinLane_arr_f_0,probWithinLane_arr_f_1,probWithinLane_arr_f_2,probWithinLane_arr_f_3,probWithinLane_arr_f_4,probCutIn_f,probCutOut_f,overlap_f,trackingTimeWithinLane_f
  Vector Concatenate : Concatenate  NumInputs=5
  TARGRTOBJECTS_ST : Outport  OutDataTypeStr=Bus: TARGETOBJECT
  wires:
  Bus Selector4/8 -> Vector Concatenate/4  "<probWithinLane_arr_f_3>"
  Bus Selector4/11 -> Bus Creator1/7  "<probCutOut_f>"
  Bus Selector4/10 -> Bus Creator1/6  "<probCutIn_f>"
  Bus Selector4/12 -> Bus Creator1/8  "<overlap_f>"
  Bus Selector4/9 -> Vector Concatenate/5  "<probWithinLane_arr_f_4>"
  Bus Selector4/2 -> Bus Creator1/2  "<TTC_f>"
  Bus Selector4/5 -> Vector Concatenate/1  "<probWithinLane_arr_f_0>"
  <LANE_3_TARGETOBJECT_0_ST>/1 -> Bus Selector4/1
  Bus Selector4/6 -> Vector Concatenate/2  "<probWithinLane_arr_f_1>"
  Bus Selector4/13 -> Bus Creator1/9  "<trackingTimeWithinLane_f>"
  Bus Selector4/1 -> Bus Creator1/1  "<dis2EgoLaneCenter>"
  Bus Selector4/7 -> Vector Concatenate/3  "<probWithinLane_arr_f_2>"
  Vector Concatenate/1 -> Bus Creator1/5
  Bus Selector4/3 -> Bus Creator1/3  "<ID_un8>"
  Bus Creator1/1 -> TARGRTOBJECTS_ST/1
  Bus Selector4/4 -> Bus Creator1/4  "<Index_un8>"

== system LM_TOS_new/LM_TOS_MODEL/adapter2/Lane_3/Subsystem9 ==
  <LANE_3_TARGETOBJECT_0_ST> : Inport
  Bus Creator1 : BusCreator  Inputs=9  OutDataTypeStr=Bus: TARGETOBJECT  NonVirtualBus=on
  Bus Selector4 : BusSelector  OutputSignals=dis2EgoLaneCenter,TTC_f,ID_un8,Index_un8,probWithinLane_arr_f_0,probWithinLane_arr_f_1,probWithinLane_arr_f_2,probWithinLane_arr_f_3,probWithinLane_arr_f_4,probCutIn_f,probCutOut_f,overlap_f,trackingTimeWithinLane_f
  Vector Concatenate : Concatenate  NumInputs=5
  TARGRTOBJECTS_ST : Outport  OutDataTypeStr=Bus: TARGETOBJECT
  wires:
  Bus Selector4/4 -> Bus Creator1/4  "<Index_un8>"
  Bus Creator1/1 -> TARGRTOBJECTS_ST/1
  Bus Selector4/3 -> Bus Creator1/3  "<ID_un8>"
  Vector Concatenate/1 -> Bus Creator1/5
  Bus Selector4/7 -> Vector Concatenate/3  "<probWithinLane_arr_f_2>"
  Bus Selector4/1 -> Bus Creator1/1  "<dis2EgoLaneCenter>"
  Bus Selector4/13 -> Bus Creator1/9  "<trackingTimeWithinLane_f>"
  Bus Selector4/6 -> Vector Concatenate/2  "<probWithinLane_arr_f_1>"
  <LANE_3_TARGETOBJECT_0_ST>/1 -> Bus Selector4/1
  Bus Selector4/5 -> Vector Concatenate/1  "<probWithinLane_arr_f_0>"
  Bus Selector4/2 -> Bus Creator1/2  "<TTC_f>"
  Bus Selector4/9 -> Vector Concatenate/5  "<probWithinLane_arr_f_4>"
  Bus Selector4/12 -> Bus Creator1/8  "<overlap_f>"
  Bus Selector4/10 -> Bus Creator1/6  "<probCutIn_f>"
  Bus Selector4/11 -> Bus Creator1/7  "<probCutOut_f>"
  Bus Selector4/8 -> Vector Concatenate/4  "<probWithinLane_arr_f_3>"

== system LM_TOS_new/LM_TOS_MODEL/adapter2/Lane_4/Subsystem ==
  <LANE_0_TARGETOBJECT_0_ST> : Inport
  Bus Creator1 : BusCreator  Inputs=9  OutDataTypeStr=Bus: TARGETOBJECT  NonVirtualBus=on
  Bus Selector4 : BusSelector  OutputSignals=dis2EgoLaneCenter,TTC_f,ID_un8,Index_un8,probWithinLane_arr_f_0,probWithinLane_arr_f_1,probWithinLane_arr_f_2,probWithinLane_arr_f_3,probWithinLane_arr_f_4,probCutIn_f,probCutOut_f,overlap_f,trackingTimeWithinLane_f
  Vector Concatenate : Concatenate  NumInputs=5
  TARGRTOBJECTS_ST : Outport  OutDataTypeStr=Bus: TARGETOBJECT
  wires:
  Bus Selector4/4 -> Bus Creator1/4  "<Index_un8>"
  Bus Creator1/1 -> TARGRTOBJECTS_ST/1
  Bus Selector4/3 -> Bus Creator1/3  "<ID_un8>"
  Vector Concatenate/1 -> Bus Creator1/5
  Bus Selector4/7 -> Vector Concatenate/3  "<probWithinLane_arr_f_2>"
  Bus Selector4/1 -> Bus Creator1/1  "<dis2EgoLaneCenter>"
  Bus Selector4/13 -> Bus Creator1/9  "<trackingTimeWithinLane_f>"
  Bus Selector4/6 -> Vector Concatenate/2  "<probWithinLane_arr_f_1>"
  <LANE_0_TARGETOBJECT_0_ST>/1 -> Bus Selector4/1
  Bus Selector4/5 -> Vector Concatenate/1  "<probWithinLane_arr_f_0>"
  Bus Selector4/2 -> Bus Creator1/2  "<TTC_f>"
  Bus Selector4/9 -> Vector Concatenate/5  "<probWithinLane_arr_f_4>"
  Bus Selector4/12 -> Bus Creator1/8  "<overlap_f>"
  Bus Selector4/10 -> Bus Creator1/6  "<probCutIn_f>"
  Bus Selector4/11 -> Bus Creator1/7  "<probCutOut_f>"
  Bus Selector4/8 -> Vector Concatenate/4  "<probWithinLane_arr_f_3>"

== system LM_TOS_new/LM_TOS_MODEL/adapter2/Lane_4/Subsystem1 ==
  <LANE_0_TARGETOBJECT_0_ST> : Inport
  Bus Creator1 : BusCreator  Inputs=9  OutDataTypeStr=Bus: TARGETOBJECT  NonVirtualBus=on
  Bus Selector4 : BusSelector  OutputSignals=dis2EgoLaneCenter,TTC_f,ID_un8,Index_un8,probWithinLane_arr_f_0,probWithinLane_arr_f_1,probWithinLane_arr_f_2,probWithinLane_arr_f_3,probWithinLane_arr_f_4,probCutIn_f,probCutOut_f,overlap_f,trackingTimeWithinLane_f
  Vector Concatenate : Concatenate  NumInputs=5
  TARGRTOBJECTS_ST : Outport  OutDataTypeStr=Bus: TARGETOBJECT
  wires:
  Bus Selector4/8 -> Vector Concatenate/4  "<probWithinLane_arr_f_3>"
  Bus Selector4/11 -> Bus Creator1/7  "<probCutOut_f>"
  Bus Selector4/10 -> Bus Creator1/6  "<probCutIn_f>"
  Bus Selector4/12 -> Bus Creator1/8  "<overlap_f>"
  Bus Selector4/9 -> Vector Concatenate/5  "<probWithinLane_arr_f_4>"
  Bus Selector4/2 -> Bus Creator1/2  "<TTC_f>"
  Bus Selector4/5 -> Vector Concatenate/1  "<probWithinLane_arr_f_0>"
  <LANE_0_TARGETOBJECT_0_ST>/1 -> Bus Selector4/1
  Bus Selector4/6 -> Vector Concatenate/2  "<probWithinLane_arr_f_1>"
  Bus Selector4/13 -> Bus Creator1/9  "<trackingTimeWithinLane_f>"
  Bus Selector4/1 -> Bus Creator1/1  "<dis2EgoLaneCenter>"
  Bus Selector4/7 -> Vector Concatenate/3  "<probWithinLane_arr_f_2>"
  Vector Concatenate/1 -> Bus Creator1/5
  Bus Selector4/3 -> Bus Creator1/3  "<ID_un8>"
  Bus Creator1/1 -> TARGRTOBJECTS_ST/1
  Bus Selector4/4 -> Bus Creator1/4  "<Index_un8>"

== system LM_TOS_new/LM_TOS_MODEL/adapter2/Lane_4/Subsystem10 ==
  <LANE_4_TARGETOBJECT_0_ST> : Inport
  Bus Creator1 : BusCreator  Inputs=7  OutDataTypeStr=Bus: SEGMENT  NonVirtualBus=on
  Bus Selector4 : BusSelector  OutputSignals=coef_arr_f_0,coef_arr_f_1,coef_arr_f_2,coef_arr_f_3,dlowerLimit_f,dupperLimit_f,numOfSegment_un8,available_b,detectedByVideo_b,quality_f
  Vector Concatenate : Concatenate  NumInputs=4
  SEGMENT_ST : Outport  OutDataTypeStr=Bus: SEGMENT
  wires:
  Bus Creator1/1 -> SEGMENT_ST/1
  <LANE_4_TARGETOBJECT_0_ST>/1 -> Bus Selector4/1
  Bus Selector4/2 -> Vector Concatenate/2  "<coef_arr_f_1>"
  Bus Selector4/1 -> Vector Concatenate/1  "<coef_arr_f_0>"
  Bus Selector4/3 -> Vector Concatenate/3  "<coef_arr_f_2>"
  Bus Selector4/4 -> Vector Concatenate/4  "<coef_arr_f_3>"
  Vector Concatenate/1 -> Bus Creator1/1
  Bus Selector4/5 -> Bus Creator1/2  "<dlowerLimit_f>"
  Bus Selector4/10 -> Bus Creator1/7  "<quality_f>"
  Bus Selector4/9 -> Bus Creator1/6  "<detectedByVideo_b>"
  Bus Selector4/8 -> Bus Creator1/5  "<available_b>"
  Bus Selector4/7 -> Bus Creator1/4  "<numOfSegment_un8>"
  Bus Selector4/6 -> Bus Creator1/3  "<dupperLimit_f>"

== system LM_TOS_new/LM_TOS_MODEL/adapter2/Lane_4/Subsystem11 ==
  <LANE_4_TARGETOBJECT_0_ST> : Inport
  Bus Creator1 : BusCreator  Inputs=7  OutDataTypeStr=Bus: SEGMENT  NonVirtualBus=on
  Bus Selector4 : BusSelector  OutputSignals=coef_arr_f_0,coef_arr_f_1,coef_arr_f_2,coef_arr_f_3,dlowerLimit_f,dupperLimit_f,numOfSegment_un8,available_b,detectedByVideo_b,quality_f
  Vector Concatenate : Concatenate  NumInputs=4
  SEGMENT_ST : Outport  OutDataTypeStr=Bus: SEGMENT
  wires:
  Bus Selector4/6 -> Bus Creator1/3  "<dupperLimit_f>"
  Bus Selector4/7 -> Bus Creator1/4  "<numOfSegment_un8>"
  Bus Selector4/8 -> Bus Creator1/5  "<available_b>"
  Bus Selector4/9 -> Bus Creator1/6  "<detectedByVideo_b>"
  Bus Selector4/10 -> Bus Creator1/7  "<quality_f>"
  Bus Selector4/5 -> Bus Creator1/2  "<dlowerLimit_f>"
  Vector Concatenate/1 -> Bus Creator1/1
  Bus Selector4/4 -> Vector Concatenate/4  "<coef_arr_f_3>"
  Bus Selector4/3 -> Vector Concatenate/3  "<coef_arr_f_2>"
  Bus Selector4/1 -> Vector Concatenate/1  "<coef_arr_f_0>"
  Bus Selector4/2 -> Vector Concatenate/2  "<coef_arr_f_1>"
  <LANE_4_TARGETOBJECT_0_ST>/1 -> Bus Selector4/1
  Bus Creator1/1 -> SEGMENT_ST/1

== system LM_TOS_new/LM_TOS_MODEL/adapter2/Lane_4/Subsystem12 ==
  <LANE_4_TARGETOBJECT_0_ST> : Inport
  Bus Creator1 : BusCreator  Inputs=7  OutDataTypeStr=Bus: SEGMENT  NonVirtualBus=on
  Bus Selector4 : BusSelector  OutputSignals=coef_arr_f_0,coef_arr_f_1,coef_arr_f_2,coef_arr_f_3,dlowerLimit_f,dupperLimit_f,numOfSegment_un8,available_b,detectedByVideo_b,quality_f
  Vector Concatenate : Concatenate  NumInputs=4
  SEGMENT_ST : Outport  OutDataTypeStr=Bus: SEGMENT
  wires:
  Bus Creator1/1 -> SEGMENT_ST/1
  <LANE_4_TARGETOBJECT_0_ST>/1 -> Bus Selector4/1
  Bus Selector4/2 -> Vector Concatenate/2  "<coef_arr_f_1>"
  Bus Selector4/1 -> Vector Concatenate/1  "<coef_arr_f_0>"
  Bus Selector4/3 -> Vector Concatenate/3  "<coef_arr_f_2>"
  Bus Selector4/4 -> Vector Concatenate/4  "<coef_arr_f_3>"
  Vector Concatenate/1 -> Bus Creator1/1
  Bus Selector4/5 -> Bus Creator1/2  "<dlowerLimit_f>"
  Bus Selector4/10 -> Bus Creator1/7  "<quality_f>"
  Bus Selector4/9 -> Bus Creator1/6  "<detectedByVideo_b>"
  Bus Selector4/8 -> Bus Creator1/5  "<available_b>"
  Bus Selector4/7 -> Bus Creator1/4  "<numOfSegment_un8>"
  Bus Selector4/6 -> Bus Creator1/3  "<dupperLimit_f>"

== system LM_TOS_new/LM_TOS_MODEL/adapter2/Lane_4/Subsystem13 ==
  <LANE_4_TARGETOBJECT_0_ST> : Inport
  Bus Creator1 : BusCreator  Inputs=7  OutDataTypeStr=Bus: SEGMENT  NonVirtualBus=on
  Bus Selector4 : BusSelector  OutputSignals=coef_arr_f_0,coef_arr_f_1,coef_arr_f_2,coef_arr_f_3,dlowerLimit_f,dupperLimit_f,numOfSegment_un8,available_b,detectedByVideo_b,quality_f
  Vector Concatenate : Concatenate  NumInputs=4
  SEGMENT_ST : Outport  OutDataTypeStr=Bus: SEGMENT
  wires:
  Bus Selector4/6 -> Bus Creator1/3  "<dupperLimit_f>"
  Bus Selector4/7 -> Bus Creator1/4  "<numOfSegment_un8>"
  Bus Selector4/8 -> Bus Creator1/5  "<available_b>"
  Bus Selector4/9 -> Bus Creator1/6  "<detectedByVideo_b>"
  Bus Selector4/10 -> Bus Creator1/7  "<quality_f>"
  Bus Selector4/5 -> Bus Creator1/2  "<dlowerLimit_f>"
  Vector Concatenate/1 -> Bus Creator1/1
  Bus Selector4/4 -> Vector Concatenate/4  "<coef_arr_f_3>"
  Bus Selector4/3 -> Vector Concatenate/3  "<coef_arr_f_2>"
  Bus Selector4/1 -> Vector Concatenate/1  "<coef_arr_f_0>"
  Bus Selector4/2 -> Vector Concatenate/2  "<coef_arr_f_1>"
  <LANE_4_TARGETOBJECT_0_ST>/1 -> Bus Selector4/1
  Bus Creator1/1 -> SEGMENT_ST/1

== system LM_TOS_new/LM_TOS_MODEL/adapter2/Lane_4/Subsystem14 ==
  <LANE_4_TARGETOBJECT_0_ST> : Inport
  Bus Creator1 : BusCreator  Inputs=7  OutDataTypeStr=Bus: SEGMENT  NonVirtualBus=on
  Bus Selector4 : BusSelector  OutputSignals=coef_arr_f_0,coef_arr_f_1,coef_arr_f_2,coef_arr_f_3,dlowerLimit_f,dupperLimit_f,numOfSegment_un8,available_b,detectedByVideo_b,quality_f
  Vector Concatenate : Concatenate  NumInputs=4
  SEGMENT_ST : Outport  OutDataTypeStr=Bus: SEGMENT
  wires:
  Bus Creator1/1 -> SEGMENT_ST/1
  <LANE_4_TARGETOBJECT_0_ST>/1 -> Bus Selector4/1
  Bus Selector4/2 -> Vector Concatenate/2  "<coef_arr_f_1>"
  Bus Selector4/1 -> Vector Concatenate/1  "<coef_arr_f_0>"
  Bus Selector4/3 -> Vector Concatenate/3  "<coef_arr_f_2>"
  Bus Selector4/4 -> Vector Concatenate/4  "<coef_arr_f_3>"
  Vector Concatenate/1 -> Bus Creator1/1
  Bus Selector4/5 -> Bus Creator1/2  "<dlowerLimit_f>"
  Bus Selector4/10 -> Bus Creator1/7  "<quality_f>"
  Bus Selector4/9 -> Bus Creator1/6  "<detectedByVideo_b>"
  Bus Selector4/8 -> Bus Creator1/5  "<available_b>"
  Bus Selector4/7 -> Bus Creator1/4  "<numOfSegment_un8>"
  Bus Selector4/6 -> Bus Creator1/3  "<dupperLimit_f>"

== system LM_TOS_new/LM_TOS_MODEL/adapter2/Lane_4/Subsystem15 ==
  <LANE_4_TARGETOBJECT_0_ST> : Inport
  Bus Creator1 : BusCreator  Inputs=7  OutDataTypeStr=Bus: SEGMENT  NonVirtualBus=on
  Bus Selector4 : BusSelector  OutputSignals=coef_arr_f_0,coef_arr_f_1,coef_arr_f_2,coef_arr_f_3,dlowerLimit_f,dupperLimit_f,numOfSegment_un8,available_b,detectedByVideo_b,quality_f
  Vector Concatenate : Concatenate  NumInputs=4
  SEGMENT_ST : Outport  OutDataTypeStr=Bus: SEGMENT
  wires:
  Bus Selector4/6 -> Bus Creator1/3  "<dupperLimit_f>"
  Bus Selector4/7 -> Bus Creator1/4  "<numOfSegment_un8>"
  Bus Selector4/8 -> Bus Creator1/5  "<available_b>"
  Bus Selector4/9 -> Bus Creator1/6  "<detectedByVideo_b>"
  Bus Selector4/10 -> Bus Creator1/7  "<quality_f>"
  Bus Selector4/5 -> Bus Creator1/2  "<dlowerLimit_f>"
  Vector Concatenate/1 -> Bus Creator1/1
  Bus Selector4/4 -> Vector Concatenate/4  "<coef_arr_f_3>"
  Bus Selector4/3 -> Vector Concatenate/3  "<coef_arr_f_2>"
  Bus Selector4/1 -> Vector Concatenate/1  "<coef_arr_f_0>"
  Bus Selector4/2 -> Vector Concatenate/2  "<coef_arr_f_1>"
  <LANE_4_TARGETOBJECT_0_ST>/1 -> Bus Selector4/1
  Bus Creator1/1 -> SEGMENT_ST/1

== system LM_TOS_new/LM_TOS_MODEL/adapter2/Lane_4/Subsystem2 ==
  <LANE_0_TARGETOBJECT_0_ST> : Inport
  Bus Creator1 : BusCreator  Inputs=9  OutDataTypeStr=Bus: TARGETOBJECT  NonVirtualBus=on
  Bus Selector4 : BusSelector  OutputSignals=dis2EgoLaneCenter,TTC_f,ID_un8,Index_un8,probWithinLane_arr_f_0,probWithinLane_arr_f_1,probWithinLane_arr_f_2,probWithinLane_arr_f_3,probWithinLane_arr_f_4,probCutIn_f,probCutOut_f,overlap_f,trackingTimeWithinLane_f
  Vector Concatenate : Concatenate  NumInputs=5
  TARGRTOBJECTS_ST : Outport  OutDataTypeStr=Bus: TARGETOBJECT
  wires:
  Bus Selector4/4 -> Bus Creator1/4  "<Index_un8>"
  Bus Creator1/1 -> TARGRTOBJECTS_ST/1
  Bus Selector4/3 -> Bus Creator1/3  "<ID_un8>"
  Vector Concatenate/1 -> Bus Creator1/5
  Bus Selector4/7 -> Vector Concatenate/3  "<probWithinLane_arr_f_2>"
  Bus Selector4/1 -> Bus Creator1/1  "<dis2EgoLaneCenter>"
  Bus Selector4/13 -> Bus Creator1/9  "<trackingTimeWithinLane_f>"
  Bus Selector4/6 -> Vector Concatenate/2  "<probWithinLane_arr_f_1>"
  <LANE_0_TARGETOBJECT_0_ST>/1 -> Bus Selector4/1
  Bus Selector4/5 -> Vector Concatenate/1  "<probWithinLane_arr_f_0>"
  Bus Selector4/2 -> Bus Creator1/2  "<TTC_f>"
  Bus Selector4/9 -> Vector Concatenate/5  "<probWithinLane_arr_f_4>"
  Bus Selector4/12 -> Bus Creator1/8  "<overlap_f>"
  Bus Selector4/10 -> Bus Creator1/6  "<probCutIn_f>"
  Bus Selector4/11 -> Bus Creator1/7  "<probCutOut_f>"
  Bus Selector4/8 -> Vector Concatenate/4  "<probWithinLane_arr_f_3>"

== system LM_TOS_new/LM_TOS_MODEL/adapter2/Lane_4/Subsystem3 ==
  <LANE_0_TARGETOBJECT_0_ST> : Inport
  Bus Creator1 : BusCreator  Inputs=9  OutDataTypeStr=Bus: TARGETOBJECT  NonVirtualBus=on
  Bus Selector4 : BusSelector  OutputSignals=dis2EgoLaneCenter,TTC_f,ID_un8,Index_un8,probWithinLane_arr_f_0,probWithinLane_arr_f_1,probWithinLane_arr_f_2,probWithinLane_arr_f_3,probWithinLane_arr_f_4,probCutIn_f,probCutOut_f,overlap_f,trackingTimeWithinLane_f
  Vector Concatenate : Concatenate  NumInputs=5
  TARGRTOBJECTS_ST : Outport  OutDataTypeStr=Bus: TARGETOBJECT
  wires:
  Bus Selector4/8 -> Vector Concatenate/4  "<probWithinLane_arr_f_3>"
  Bus Selector4/11 -> Bus Creator1/7  "<probCutOut_f>"
  Bus Selector4/10 -> Bus Creator1/6  "<probCutIn_f>"
  Bus Selector4/12 -> Bus Creator1/8  "<overlap_f>"
  Bus Selector4/9 -> Vector Concatenate/5  "<probWithinLane_arr_f_4>"
  Bus Selector4/2 -> Bus Creator1/2  "<TTC_f>"
  Bus Selector4/5 -> Vector Concatenate/1  "<probWithinLane_arr_f_0>"
  <LANE_0_TARGETOBJECT_0_ST>/1 -> Bus Selector4/1
  Bus Selector4/6 -> Vector Concatenate/2  "<probWithinLane_arr_f_1>"
  Bus Selector4/13 -> Bus Creator1/9  "<trackingTimeWithinLane_f>"
  Bus Selector4/1 -> Bus Creator1/1  "<dis2EgoLaneCenter>"
  Bus Selector4/7 -> Vector Concatenate/3  "<probWithinLane_arr_f_2>"
  Vector Concatenate/1 -> Bus Creator1/5
  Bus Selector4/3 -> Bus Creator1/3  "<ID_un8>"
  Bus Creator1/1 -> TARGRTOBJECTS_ST/1
  Bus Selector4/4 -> Bus Creator1/4  "<Index_un8>"
